simulink model "LQR_Model"  (R2016b)
settings: Solver=ode45  StartTime=0.0  StopTime=60  RelTol=1e-3  EnableMultiTasking=on
values from neighbouring files (symbols this model uses):
  B = [0 0 ... (first row only)    [lin_discr_model.m]
  C = [1 0 0 0 ... (first row only)    [lin_discr_model.m]
  L = place(A_eq1_d',C_eq1_d',pdes)'    [lin_discr_model.m]
undefined symbols (not defined in the file or in its folder): A, adingain, adinoffs, Amp, daoutgain, daoutoffs, Freq, K_lq, x_op
undefined symbols (not defined in the file): h
settings Model: Creator=rbabuska  LastModifiedBy=jkleinschiphor
settings DataIOCC: LimitDataPoints=on  SaveFormat=Array  SignalLoggingName=sigsOut
settings OptimizationCC: BooleanDataType=off  ExpressionDepthLimit=2147483647  InitFltsAndDblsToZero=on  LifeSpan=inf
settings DebuggingCC: SaveWithParameterizedLinksMsg=none  SignalResolutionControl=TryResolveAllWithWarning  MultiTaskDSMMsg=warning  MultiTaskCondExecSysMsg=none  AllowSymbolicDim=off  StateNameClashWarn=warning  SFUnexpectedBacktrackingDiag=warning  SFNoUnconditionalDefaultTransitionDiag=warning  SFExecutionAtInitializationDiag=none
settings HardwareCC: ProdBitPerPointer=32  ProdBitPerSizeT=32  ProdBitPerPtrDiffT=32  ProdLargestAtomicFloat=None  ProdIntDivRoundTo=Undefined  ProdEndianess=Unspecified  ProdWordSize=32  ProdHWDeviceType=32-bit Generic  TargetUnknown=on
settings ModelReferenceCC: PropagateSignalLabelsOutOfModel=off
settings GRTTargetCC: TargetFcnLib=ansi_tfl_tmw.mat  TargetLangStandard=C89/C90 (ANSI)  GeneratePreprocessorConditionals=Disable all  CombineOutputUpdateFcns=off  GRTInterface=on
settings ConfigComp: CovMetricSettings=dw  CovHtmlReporting=on  CovSaveCumulativeToWorkspaceVar=on  CovSaveSingleToWorkspaceVar=on  CovExternalEMLEnable=off

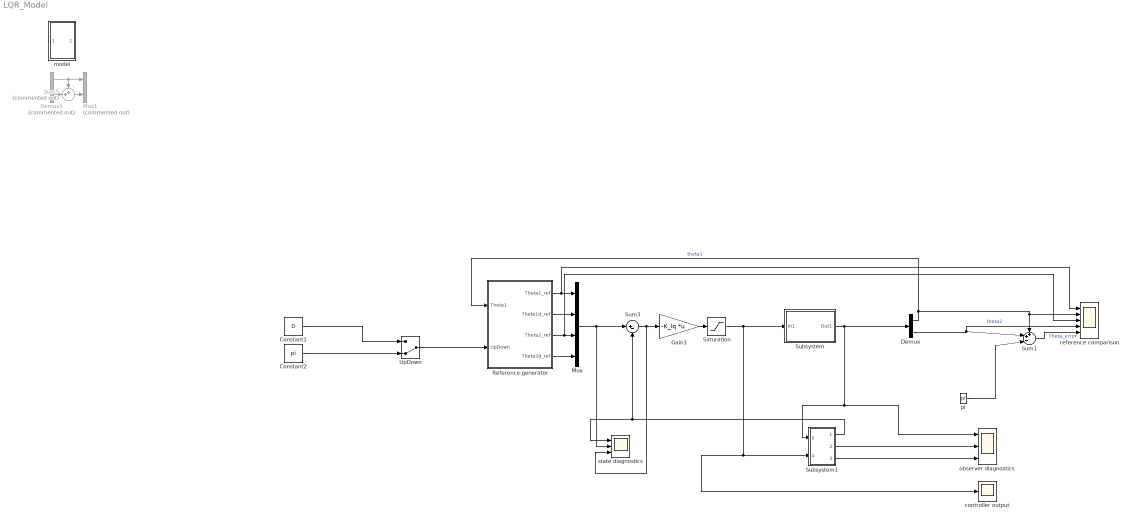
== system LQR_Model ==
  Constant1 : Constant  Value=0
  Constant2 : Constant  Value=pi
  Demux : Demux  Outputs=2
  Demux1 : Demux  Commented=on  Outputs=2
  Gain3 : Gain  Gain=-K_lq  Multiplication=Matrix(K*u)
  Mux : Mux
  Mux1 : Mux  Commented=on  Inputs=2
  "Reference generator " : Subsystem
  Saturation : Saturate  UpperLimit=1  LowerLimit=-1
  Subsystem : Subsystem
      mask Display: disp('Rotational\nPendulum')
  Subsystem1 : Subsystem
  Sum1 : Sum  Inputs=++-|
  Sum3 : Sum  Inputs=|+-
  Sum5 : Sum  Commented=on  Inputs=++|
  UpDown : ManualSwitch  CurrentSetting=0
  controller output : Scope
  model : Subsystem
  observer diagnostics : Scope  NumInputPorts=3
  pi : Constant  Value=pi
  reference comparison : Scope  NumInputPorts=5
  state diagnostics : Scope  NumInputPorts=3
  wires:
  Demux/1 -> reference comparison/2, Sum1/1, "Reference generator "/1(Theta1)  "theta1"
  Demux/2 -> Sum1/2, reference comparison/4  "theta2"
  Sum3/1 -> state diagnostics/3, Gain3/1
  Saturation/1 -> controller output/1, Subsystem1/2(u), Subsystem/1(In1)
  Gain3/1 -> Saturation/1
  Demux1/1 -> Sum5/1, Mux1/1
  Demux1/2 -> Sum5/2
  Sum5/1 -> Mux1/2
  Subsystem/1(Out1) -> Subsystem1/1(y), observer diagnostics/1, Demux/1
  Subsystem1/1(x_hat) -> state diagnostics/1, Sum3/2
  Subsystem1/2(y_hat) -> observer diagnostics/2
  Subsystem1/3(y_err) -> observer diagnostics/3
  Mux/1 -> state diagnostics/2, Sum3/1
  Sum1/1 -> reference comparison/5  "Theta_error"
  pi/1 -> Sum1/3
  Constant1/1 -> UpDown/1
  Constant2/1 -> UpDown/2
  "Reference generator "/1(Theta1_ref) -> reference comparison/1, Mux/1
  "Reference generator "/3(Theta2_ref) -> reference comparison/3, Mux/3
  UpDown/1 -> "Reference generator "/2(UpDown)
  "Reference generator "/2(Theta1d_ref) -> Mux/2
  "Reference generator "/4(Theta2d_ref) -> Mux/4

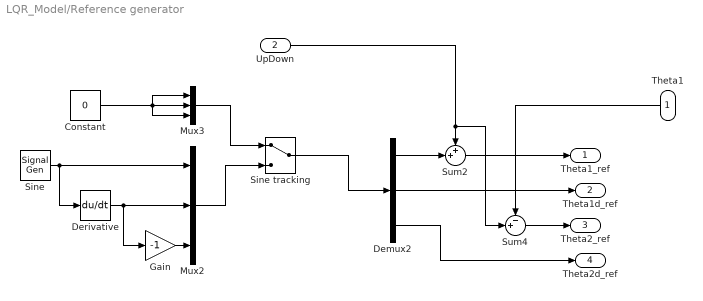
== system LQR_Model/Reference generator  ==
  Theta1 : Inport
  UpDown : Inport  Port=2
  Constant : Constant  Value=0
  Demux2 : Demux  Outputs=3
  Derivative : Derivative
  Gain : Gain  Gain=-1
  Mux2 : Mux  Inputs=3
  Mux3 : Mux  Inputs=3
  Sine : SignalGenerator  Amplitude=Amp  Frequency=Freq
  Sine tracking : ManualSwitch
  Sum2 : Sum  Inputs=++|
  Sum4 : Sum  Inputs=-+|
  Theta1_ref : Outport
  Theta1d_ref : Outport  Port=2
  Theta2_ref : Outport  Port=3
  Theta2d_ref : Outport  Port=4
  wires:
  Demux2/2 -> Theta1d_ref/1
  Sine/1 -> Derivative/1, Mux2/1
  Derivative/1 -> Gain/1, Mux2/2
  Demux2/3 -> Theta2d_ref/1
  Sum4/1 -> Theta2_ref/1
  UpDown/1 -> Sum4/2, Sum2/1
  Sine tracking/1 -> Demux2/1
  Gain/1 -> Mux2/3
  Mux3/1 -> Sine tracking/1
  Constant/1 -> Mux3/3, Mux3/1, Mux3/2
  Mux2/1 -> Sine tracking/2
  Demux2/1 -> Sum2/2
  Theta1/1 -> Sum4/1
  Sum2/1 -> Theta1_ref/1

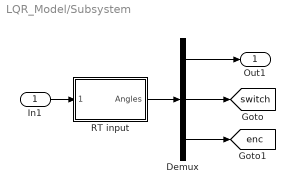
== system LQR_Model/Subsystem ==
  In1 : Inport
  Demux : Demux  Outputs=[2 4 1]
  RT input : Subsystem  mask{Ts=h, channels=[6 7]}
      mask prompts: Ts "Sample time [s]:"; channels "Channels to read (e.g., [6 7])"
      mask init:
      | hwinit;
      | 
      | % initialize FPGA
      | fugihandle = fugiboard('Open', 'Pendulum1');
      | fugihandle.WatchdogTimeout = 0.5;
      | fugiboard('SetParams', fugihandle);
      | fugiboard('Write', fugihandle, 0, 0, 0, 0);  % dummy write to sync interface board
      | fugiboard('Write', fugihandle, 5, 1, 0, 0);  % reset position, activate relay
      | data = fugiboard('Read', fugihandle);        % get version info from FPGA
      | % model = bitshift(data(1), -5); 
      | % version = bitand(data(1), 31);
      | % disp(sprintf('FPGA setup %d, version %d', model, version)); % for the B&P it should say 1 1, or else there is a problem
      | fugiboard('Write', fugihandle, 0, 1, 0, 0);  % end reset
      | pause(0.1);                         % give relay some time to respond
      mask Display: disp('Rotational\nPendulum')
  Out1 : Outport
  tag scope: enc=global, switch=global
  wires:
  RT input/1(Angles) -> Demux/1
  Demux/1 -> Out1/1
  Demux/2 -> [switch]
  Demux/3 -> [enc]
  In1/1 -> RT input/1(Motors)

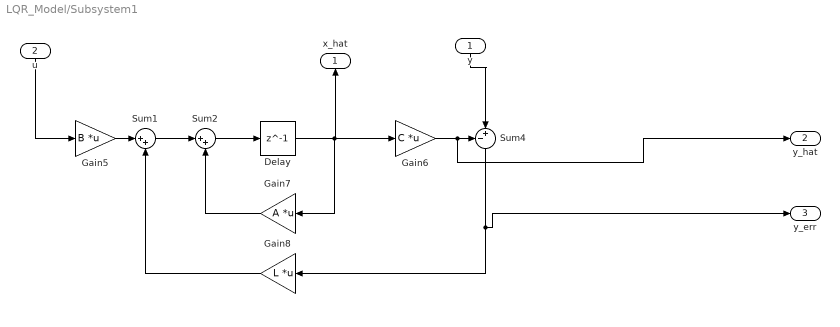
== system LQR_Model/Subsystem1 ==
  y : Inport
  u : Inport  Port=2
  Delay : Delay  DelayLength=1  InitialCondition=x_op
  Gain5 : Gain  Gain=B  Multiplication=Matrix(K*u)
  Gain6 : Gain  Gain=C  Multiplication=Matrix(K*u)
  Gain7 : Gain  Gain=A  Multiplication=Matrix(K*u)
  Gain8 : Gain  Gain=L  Multiplication=Matrix(K*u)
  Sum1 : Sum  Inputs=|++
  Sum2 : Sum  Inputs=|++
  Sum4 : Sum  Inputs=-+|
  x_hat : Outport
  y_hat : Outport  Port=2
  y_err : Outport  Port=3
  wires:
  Delay/1 -> x_hat/1, Gain6/1, Gain7/1
  Sum2/1 -> Delay/1
  Gain7/1 -> Sum2/2
  Gain6/1 -> y_hat/1, Sum4/1
  Gain8/1 -> Sum1/2
  Sum4/1 -> y_err/1, Gain8/1
  Sum1/1 -> Sum2/1
  Gain5/1 -> Sum1/1
  y/1 -> Sum4/2
  u/1 -> Gain5/1

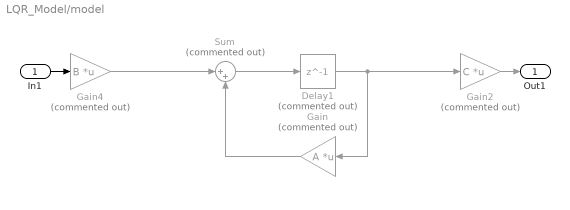
== system LQR_Model/model ==
  In1 : Inport
  Delay1 : Delay  Commented=on  DelayLength=1  InitialCondition=x_op
  Gain : Gain  Commented=on  Gain=A  Multiplication=Matrix(K*u)
  Gain2 : Gain  Commented=on  Gain=C  Multiplication=Matrix(K*u)
  Gain4 : Gain  Commented=on  Gain=B  Multiplication=Matrix(K*u)
  Sum : Sum  Commented=on  Inputs=|++
  Out1 : Outport
  wires:
  Gain4/1 -> Sum/1
  Delay1/1 -> Gain/1, Gain2/1
  Gain/1 -> Sum/2
  Sum/1 -> Delay1/1
  Gain2/1 -> Out1/1
  In1/1 -> Gain4/1

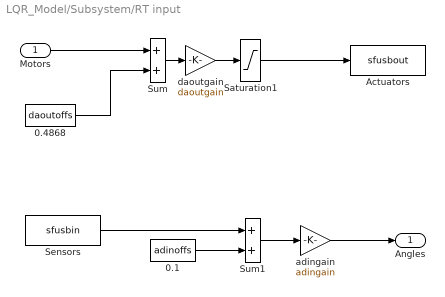
== system LQR_Model/Subsystem/RT input ==
  Motors : Inport
  0.1 : Constant  Value=adinoffs
  0.4868 : Constant  Value=daoutoffs
  Actuators : S-Function  FunctionName=sfusbout  Parameters=Ts, fugihandle  SFunctionDeploymentMode=off  EnableBusSupport=off
  Saturation1 : Saturate  UpperLimit=10  LowerLimit=-10
  Sensors : S-Function  FunctionName=sfusbin  Parameters=Ts, fugihandle, channels  SFunctionDeploymentMode=off  EnableBusSupport=off
  Sum : Sum  SaturateOnIntegerOverflow=on  InputSameDT=on  OutDataTypeStr=Inherit: Same as first input
  Sum1 : Sum  SaturateOnIntegerOverflow=on  InputSameDT=on  OutDataTypeStr=Inherit: Same as first input
  adingain : Gain  Gain=adingain  SaturateOnIntegerOverflow=on  OutDataTypeStr=Inherit: Same as input  ParamDataTypeStr=Inherit: Same as input
  daoutgain : Gain  Gain=daoutgain  SaturateOnIntegerOverflow=on  OutDataTypeStr=Inherit: Same as input  ParamDataTypeStr=Inherit: Same as input
  Angles : Outport
  wires:
  Sum/1 -> daoutgain/1
  0.4868/1 -> Sum/2
  Motors/1 -> Sum/1
  Sum1/1 -> adingain/1
  0.1/1 -> Sum1/2
  adingain/1 -> Angles/1
  Saturation1/1 -> Actuators/1
  daoutgain/1 -> Saturation1/1
  Sensors/1 -> Sum1/1
